simulink model "plantaV1"  (R2022b)
settings: Solver=VariableStepAuto  StartTime=0.0  StopTime=10.0  RelTol=1e-3
undefined symbols (not defined in the file or in its folder): b, d1, d2, Gden, Gnum, thetap, wb, wcp, wm
settings Model: Creator=felip  LastModifiedBy=felip

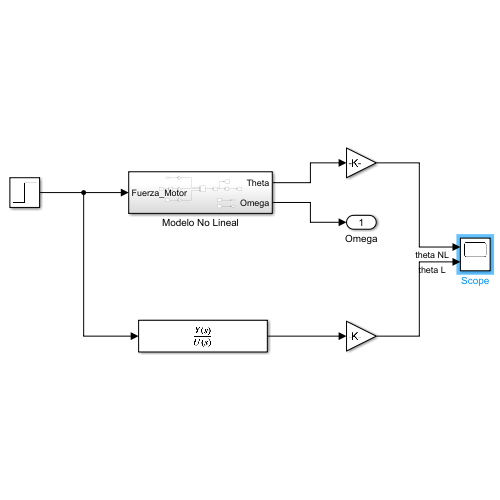
[thumbnail: Simulink's stored preview of the top-level diagram]
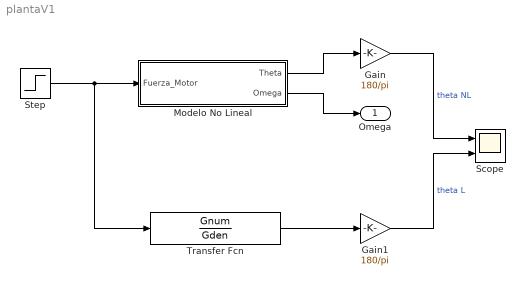
== system plantaV1 ==
  Gain : Gain  Gain=180/pi
  Gain1 : Gain  Gain=180/pi
  Modelo No Lineal : Subsystem
  Scope : Scope  NumInputPorts=2
  Step : Step  SampleTime=0
  Transfer Fcn : TransferFcn  Numerator=Gnum  Denominator=Gden
  Omega : Outport
  wires:
  Step/1 -> Transfer Fcn/1, Modelo No Lineal/1(Fuerza_Motor)
  Modelo No Lineal/1(Theta) -> Gain/1
  Modelo No Lineal/2(Omega) -> Omega/1
  Transfer Fcn/1 -> Gain1/1
  Gain/1 -> Scope/1  "theta NL"
  Gain1/1 -> Scope/2  "theta L"

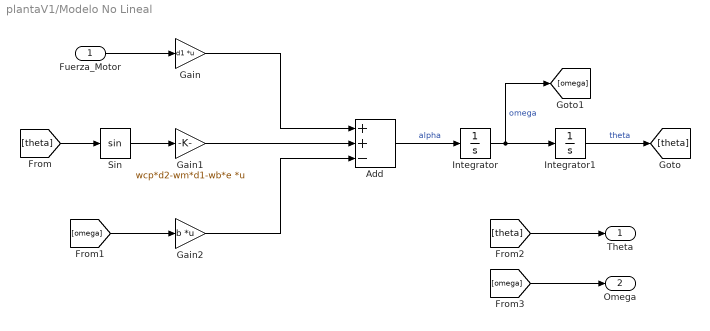
== system plantaV1/Modelo No Lineal ==
  Fuerza_Motor : Inport
  Add : Sum  Inputs=++-
  Gain : Gain  Gain=d1  Multiplication=Matrix(K*u)
  Gain1 : Gain  Gain=wcp*d2-wm*d1-wb*e  Multiplication=Matrix(K*u)
  Gain2 : Gain  Gain=b  Multiplication=Matrix(K*u)
  Integrator : Integrator
  Integrator1 : Integrator  InitialCondition=thetap*pi/180
  Sin : Trigonometry
  Theta : Outport
  Omega : Outport  Port=2
  wires:
  [omega] -> Omega/1
  Gain1/1 -> Add/2
  Integrator/1 -> [omega], Integrator1/1  "omega"
  Fuerza_Motor/1 -> Gain/1
  Integrator1/1 -> [theta]  "theta"
  Gain2/1 -> Add/3
  Gain/1 -> Add/1
  Add/1 -> Integrator/1  "alpha"
  [theta] -> Sin/1
  [omega] -> Gain2/1
  [theta] -> Theta/1
  Sin/1 -> Gain1/1
